simulink model "Lab42"  (R2023b)
settings: Solver=VariableStepAuto  StartTime=0.0  StopTime=0.5  RelTol=1e-3
libraries: spsDetailedThyristorLib x4, spsVoltageMeasurementLib x3, spsCurrentMeasurementLib x2, spsACVoltageSourceLib x1, spsControlledCurrentSourceLib x1, spsMeanLib x1, spsRMSLib x1, sps_lib x1
settings Model: Creator=niran  LastModifiedBy=niran
settings DataIOCC: ReturnWorkspaceOutputs=off

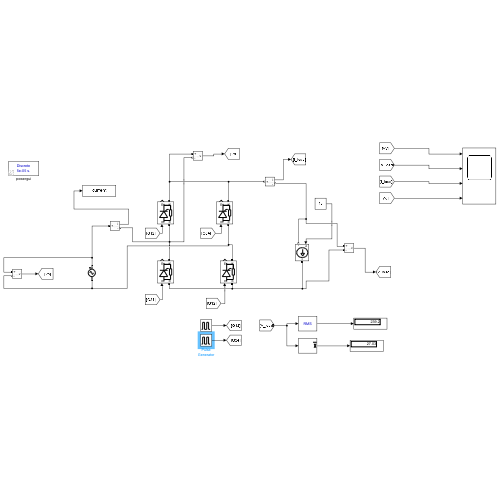
[thumbnail: Simulink's stored preview of the top-level diagram]
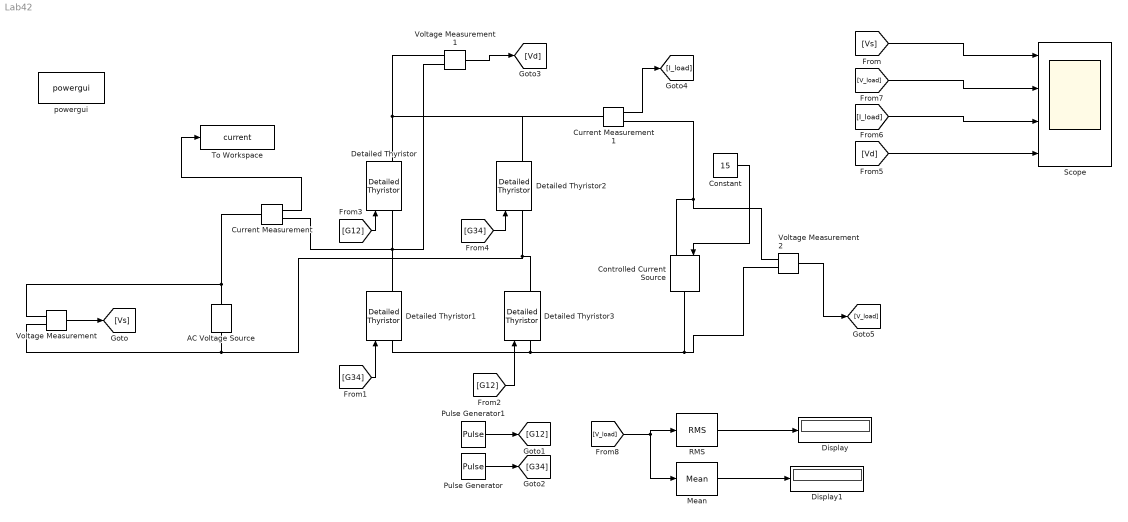
== system Lab42 ==
  AC Voltage Source : spsACVoltageSourceLib/AC Voltage Source  Amplitude=325  Phase=0  Frequency=50  SampleTime=0  Measurements=Voltage  BusType=swing  Pref=10e3  Qref=0  Qmin=-inf  Qmax=+inf
  Constant : Constant  Value=15
  Controlled Current Source : spsControlledCurrentSourceLib/Controlled Current Source  Initialize=on  Source_Type=DC  Amplitude=1  Phase=0  Frequency=0  Measurements=Current
  Current Measurement : spsCurrentMeasurementLib/Current Measurement  PhasorSimulation=off  OutputType=Complex  PSBequivalent=0
  Current Measurement1 : spsCurrentMeasurementLib/Current Measurement  PhasorSimulation=off  OutputType=Complex  PSBequivalent=0
  Detailed Thyristor{,1..3} (4 alike) : spsDetailedThyristorLib/Detailed Thyristor  Ron=0.001  Lon=1e-3  Vf=0.8  IL=0.1  Tq=100e-6  IC=0  Rs=500  Cs=250e-9  Measurements=on
      settings: LibrarySourceBlock=sps_lib/Power Electronics/Detailed Thyristor
  Display : Display
  Display1 : Display
  Mean : spsMeanLib/Mean  Freq=60  Vinit=0  Ts=0
  Pulse Generator : DiscretePulseGenerator  PulseType=Time based  Period=0.02  PulseWidth=5  PhaseDelay=0.02*(90+180)/360
  Pulse Generator1 : DiscretePulseGenerator  PulseType=Time based  Period=0.02  PulseWidth=5  PhaseDelay=90*0.02/360
  RMS : spsRMSLib/RMS  TrueRMS=on  Freq=60  RMSInit=120  Ts=0
  Scope : Scope  NumInputPorts=4
  To Workspace : ToWorkspace  VariableName=current  SaveFormat=Timeseries  SampleTime=-1
  Voltage Measurement : spsVoltageMeasurementLib/Voltage Measurement  PhasorSimulation=off  OutputType=Complex  PSBequivalent=0
  Voltage Measurement1 : spsVoltageMeasurementLib/Voltage Measurement  PhasorSimulation=off  OutputType=Complex  PSBequivalent=0
  Voltage Measurement2 : spsVoltageMeasurementLib/Voltage Measurement  PhasorSimulation=off  OutputType=Complex  PSBequivalent=0
  powergui : sps_lib/powergui  Priority=1  SimulationMode=Discrete  SampleTime=50e-6  frequency=60  Iterations=50  frequencyindice=50  Pbase=100e6  ErrMax=1e-4  UnitsV=kV  UnitsW=MW  buscounter=0  FunctionMessages=off  echomessages=off  EnableUseOfTLC=off  CurrentSourceSwitches=off  DisableSnubberDevices=off  DisableRonSwitches=off  DisableVfSwitches=off  DisplayEquations=off  AutomaticDiscreteSolvers=off  SolverType=Tustin/Backward Euler (TBE)  Interpol=off  ExternalGateDelay=off  methode=off  Ts=100  x0status=blocks  SPID=on  SwTol=0  HookPort=off  NonlinearTolerance=1e-4  nMaxIteration=100  ContinueOnMaxIteration=off  RestoreLinks=warning  ResistiveCurrentMeasurement=off  Frange=[0:2:500]  Ylog=off  Xlog=on  ShowGrid=off  save=off  variable=ZData  structure=0  ZoomFFT=off  StartTime=0.0  cycles=1  DisplayStyle=1  fundamental=60  FreqAxis=off  MaxFrequency=1000  frequencyindicesteady=1  RmsSteady=1  display=off
  wires:
  Voltage Measurement/1 -> [Vs]
  Current Measurement/1 -> To Workspace/1
  [G34] -> Detailed Thyristor1/1
  [G12] -> Detailed Thyristor3/1
  [G12] -> Detailed Thyristor/1
  [G34] -> Detailed Thyristor2/1
  Voltage Measurement1/1 -> [Vd]
  Current Measurement1/1 -> [I_load]
  Voltage Measurement2/1 -> [V_load]
  Pulse Generator1/1 -> [G12]
  Pulse Generator/1 -> [G34]
  [V_load] -> Mean/1, RMS/1
  RMS/1 -> Display/1
  Mean/1 -> Display1/1
  [V_load] -> Scope/2
  [I_load] -> Scope/3
  [Vd] -> Scope/4
  [Vs] -> Scope/1
  Constant/1 -> Controlled Current Source/1
  connections:
  AC Voltage Source/RConn1 -- Current Measurement/LConn1 -- Voltage Measurement/LConn1
  Detailed Thyristor/RConn1 -- Detailed Thyristor2/RConn1 -- Current Measurement1/LConn1 -- Voltage Measurement1/LConn1
  Voltage Measurement/LConn2 -- Detailed Thyristor3/RConn1 -- Detailed Thyristor2/LConn1 -- AC Voltage Source/LConn1
  Voltage Measurement2/LConn1 -- Controlled Current Source/LConn1 -- Current Measurement1/RConn1
  Voltage Measurement1/LConn2 -- Detailed Thyristor/LConn1 -- Detailed Thyristor1/RConn1 -- Current Measurement/RConn1
  Voltage Measurement2/LConn2 -- Controlled Current Source/RConn1 -- Detailed Thyristor1/LConn1 -- Detailed Thyristor3/LConn1
